simulink model "taller1_uav"  (R2026a)
settings: Solver=ode45  StopTime=t_final
InitFcn:
  | run('/home/sergio/Escritorio/tdc/taller1/init_taller1_simulink.m')
undefined symbols (not defined in the file or in its folder): A_full, B_full, C_sim, cas_pi_phi_den, cas_pi_phi_num, cas_pi_theta_den, cas_pi_theta_num, control_mode, D_sim, dist_amp, dist_freq, Kphi_A, Kphi_B, Kphi_C, Kphi_D, Ktheta_A, Ktheta_B, Ktheta_C, Ktheta_D, Kyaw_A, Kyaw_B, Kyaw_C, Kyaw_D, noise_sample_time, noise_var_phi, noise_var_theta, sas_D_p, sas_D_q, t_step, umax
settings Model: Creator=sergio  LastModifiedBy=sergio

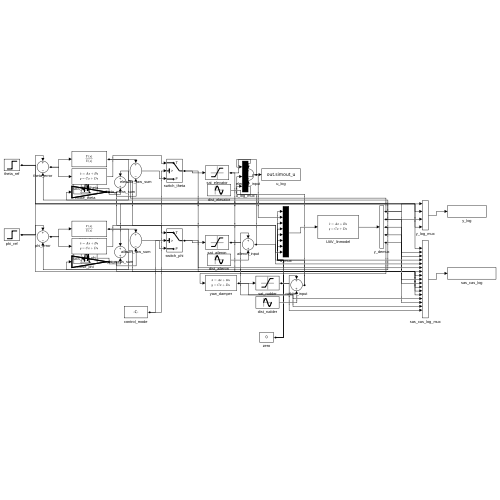
[thumbnail: Simulink's stored preview of the top-level diagram]
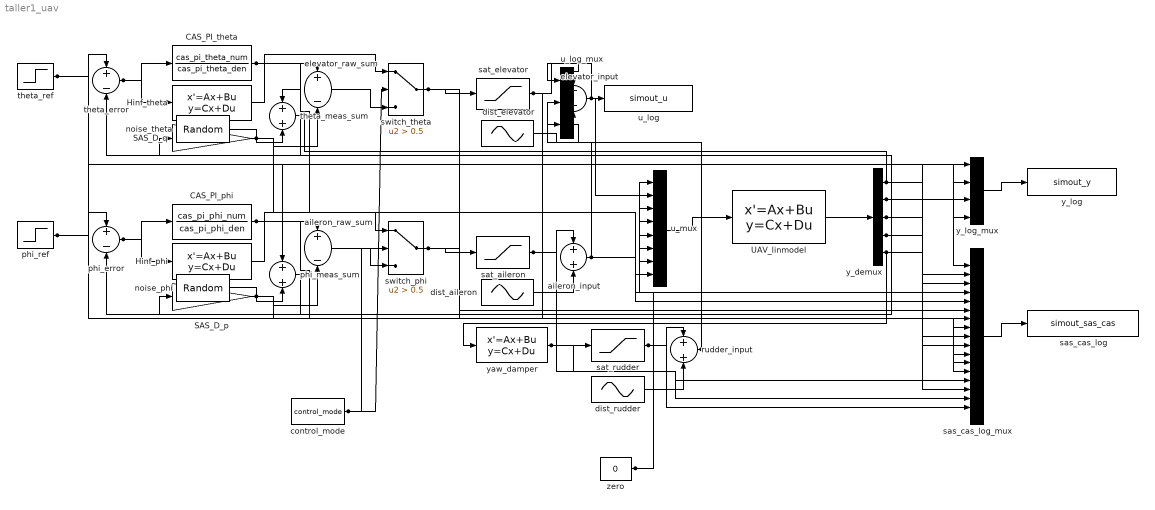
== system taller1_uav ==
  CAS_PI_phi : TransferFcn  Numerator=cas_pi_phi_num  Denominator=cas_pi_phi_den
  CAS_PI_theta : TransferFcn  Numerator=cas_pi_theta_num  Denominator=cas_pi_theta_den
  Hinf_phi : StateSpace  A=Kphi_A  B=Kphi_B  C=Kphi_C  D=Kphi_D  InitialCondition=zeros(size(Kphi_A,1),1)
  Hinf_theta : StateSpace  A=Ktheta_A  B=Ktheta_B  C=Ktheta_C  D=Ktheta_D  InitialCondition=zeros(size(Ktheta_A,1),1)
  SAS_D_p : Gain  Gain=sas_D_p
  SAS_D_q : Gain  Gain=sas_D_q
  UAV_linmodel : StateSpace  A=A_full  B=B_full  C=C_sim  D=D_sim  InitialCondition=zeros(size(A_full,1),1)
  aileron_input : Sum
  aileron_raw_sum : Sum  Inputs=+-
  control_mode : Constant  Value=control_mode
  dist_aileron : Sin  Amplitude=dist_amp  Frequency=dist_freq  Phase=pi/4  SampleTime=0
  dist_elevator : Sin  Amplitude=dist_amp  Frequency=dist_freq  SampleTime=0
  dist_rudder : Sin  Amplitude=dist_amp  Frequency=dist_freq  Phase=pi/2  SampleTime=0
  elevator_input : Sum
  elevator_raw_sum : Sum  Inputs=+-
  noise_phi : RandomNumber  Variance=noise_var_phi  Seed=17  SampleTime=noise_sample_time
  noise_theta : RandomNumber  Variance=noise_var_theta  Seed=11  SampleTime=noise_sample_time
  phi_error : Sum  Inputs=+-
  phi_meas_sum : Sum
  phi_ref : Step  Time=t_step  FinalValue=phi_ref_step  SampleTime=0
  rudder_input : Sum
  sas_cas_log : ToWorkspace  VariableName=simout_sas_cas  SaveFormat=Structure With Time  SampleTime=-1
  sas_cas_log_mux : Mux  Inputs=17
  sat_aileron : Saturate  UpperLimit=umax  LowerLimit=-umax
  sat_elevator : Saturate  UpperLimit=umax  LowerLimit=-umax
  sat_rudder : Saturate  UpperLimit=umax  LowerLimit=-umax
  switch_phi : Switch  Criteria=u2 > Threshold  Threshold=0.5  SaturateOnIntegerOverflow=off  InputSameDT=off
  switch_theta : Switch  Criteria=u2 > Threshold  Threshold=0.5  SaturateOnIntegerOverflow=off  InputSameDT=off
  theta_error : Sum  Inputs=+-
  theta_meas_sum : Sum
  theta_ref : Step  Time=t_step  FinalValue=theta_ref_step  SampleTime=0
  u_log : ToWorkspace  VariableName=simout_u  SaveFormat=Structure With Time  SampleTime=-1
  u_log_mux : Mux  Inputs=3
  u_mux : Mux  Inputs=8
  y_demux : Demux  Outputs=5
  y_log : ToWorkspace  VariableName=simout_y  SaveFormat=Structure With Time  SampleTime=-1
  y_log_mux : Mux
  yaw_damper : StateSpace  A=Kyaw_A  B=Kyaw_B  C=Kyaw_C  D=Kyaw_D  InitialCondition=0
  zero : Constant  Value=0
  wires:
  UAV_linmodel/1 -> y_demux/1
  u_mux/1 -> UAV_linmodel/1
  y_demux/1 -> theta_meas_sum/1, y_log_mux/1, sas_cas_log_mux/2
  noise_theta/1 -> theta_meas_sum/2
  theta_ref/1 -> theta_error/1, y_log_mux/2, sas_cas_log_mux/1
  theta_meas_sum/1 -> theta_error/2
  theta_error/1 -> CAS_PI_theta/1, Hinf_theta/1
  y_demux/4 -> SAS_D_q/1, sas_cas_log_mux/3
  CAS_PI_theta/1 -> elevator_raw_sum/1, sas_cas_log_mux/4
  SAS_D_q/1 -> elevator_raw_sum/2, sas_cas_log_mux/5
  Hinf_theta/1 -> switch_theta/1
  control_mode/1 -> switch_theta/2, switch_phi/2
  elevator_raw_sum/1 -> switch_theta/3
  switch_theta/1 -> sat_elevator/1, sas_cas_log_mux/6
  sat_elevator/1 -> elevator_input/1, sas_cas_log_mux/7
  dist_elevator/1 -> elevator_input/2
  y_demux/2 -> phi_meas_sum/1, y_log_mux/3, sas_cas_log_mux/9
  noise_phi/1 -> phi_meas_sum/2
  phi_ref/1 -> phi_error/1, y_log_mux/4, sas_cas_log_mux/8
  phi_meas_sum/1 -> phi_error/2
  phi_error/1 -> CAS_PI_phi/1, Hinf_phi/1
  y_demux/3 -> SAS_D_p/1, sas_cas_log_mux/10
  CAS_PI_phi/1 -> aileron_raw_sum/1, sas_cas_log_mux/11
  SAS_D_p/1 -> aileron_raw_sum/2, sas_cas_log_mux/12
  Hinf_phi/1 -> switch_phi/1
  aileron_raw_sum/1 -> switch_phi/3
  switch_phi/1 -> sat_aileron/1, sas_cas_log_mux/13
  sat_aileron/1 -> aileron_input/1, sas_cas_log_mux/14
  dist_aileron/1 -> aileron_input/2
  y_demux/5 -> yaw_damper/1, sas_cas_log_mux/15
  yaw_damper/1 -> sat_rudder/1, sas_cas_log_mux/16
  sat_rudder/1 -> rudder_input/1, sas_cas_log_mux/17
  dist_rudder/1 -> rudder_input/2
  zero/1 -> u_mux/1, u_mux/4, u_mux/5, u_mux/6, u_mux/7
  elevator_input/1 -> u_mux/2, u_log_mux/1
  rudder_input/1 -> u_mux/3, u_log_mux/3
  aileron_input/1 -> u_mux/8, u_log_mux/2
  y_log_mux/1 -> y_log/1
  u_log_mux/1 -> u_log/1
  sas_cas_log_mux/1 -> sas_cas_log/1
